simulink model "junction_cycle"  (Simulink 5.0)
settings: Solver=FixedStepDiscrete  StartTime=0.0  StopTime=10.0  RelTol=1e-3
settings Model: Creator=sofronis  LastModifiedBy=sofronis  ExtModeAutoUpdateStatusClock=off  AlgebraicLoopMsg=error

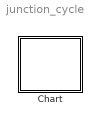
== system junction_cycle ==
  Chart : Stateflow chart

== stateflow chart Chart ==
  (junction 3) -> (junction 4) : [true]
  (junction 4) -> (junction 5) : [true]
  (junction 5) -> (junction 3) : [true]
  (junction 3) -> (junction 6)
  (junction 4) -> (junction 6)
  (junction 5) -> (junction 6)
  (default) -> (junction 3)
  data: true constant =1
